simulink model "LHC_18kW_v8"  (R2015a)
settings: Solver=ode15s  StartTime=0.0  StopTime=1e4  RelTol=1e-3
libraries: simCryogenics_lib x152, nesl_utility x108, fl_lib x15
(part 1 of 2)
settings Model: Creator=SK248285  LastModifiedBy=FB229602
settings SimscapeCC: SimscapeLogType=all  SimscapeLogLimitData=off

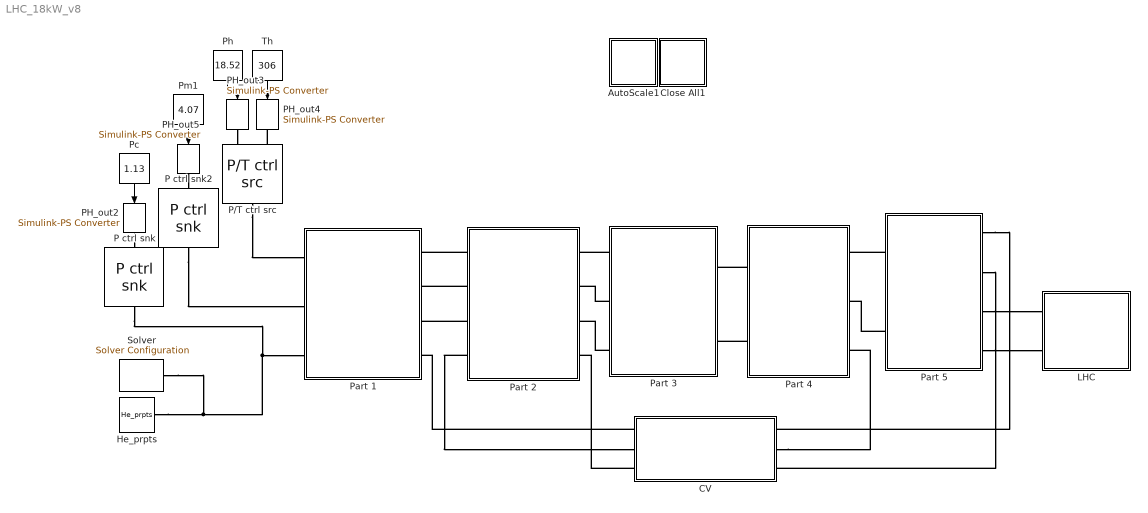
== system LHC_18kW_v8 ==
  AutoScale1 : Subsystem
      settings: OpenFcn=|
      | set(0, 'showhiddenhandles', 'on')
      | 
      | scope = findobj(0, 'Tag', 'SIMULINK_SIMSCOPE_FIGURE');
      | 
      | for i=1:length(scope)
      |   simscope('ScopeBar', 'ActionIcon', 'Find',     scope(i))
      | end
      | 
      | set(0, 'showhiddenhandles', 'off')
      mask Display: disp('Auto\nScale\nScope')
  CV : Subsystem
  Close All1 : Subsystem
      settings: OpenFcn=|
      | set(0, 'showhiddenhandles', 'on')
      | scope = findobj(0, 'Tag','SIMULINK_SIMSCOPE_FIGURE');
      | close(scope)
      | set(0, 'showhiddenhandles', 'off')
      mask Display: disp('Close\nAll\nScope')
  He_prpts : simCryogenics_lib/Utilities/He_prpts  P_min=0.01 bar  T_min=1.8 K  T_max=320 K  P_max=20 bar  Mol=4.0026 * 10 ^ (- 3) kg/mol
  LHC : Subsystem
  P ctrl snk : simCryogenics_lib/Sources_Sinks/P ctrl snk
  P ctrl snk2 : simCryogenics_lib/Sources_Sinks/P ctrl snk
  P/T ctrl src : simCryogenics_lib/Sources_Sinks/P//T ctrl src
  PH_out2 : nesl_utility/Simulink-PS Converter  PhysicalDomain=network_engine_domain  SubClassName=ps_input  LeftPortType=input  RightPortType=output  PseudoPeriodic=off  Frequencies=[]  NoiseDistribution=none  NoiseParameters=[]  Unit=bar  AffineConversion=off  InputFiltering=off  SimscapeFilterOrder=1  InputFilterTimeConstant=0.001  UdotUserProvided=1
  PH_out3 : nesl_utility/Simulink-PS Converter  PhysicalDomain=network_engine_domain  SubClassName=ps_input  LeftPortType=input  RightPortType=output  PseudoPeriodic=off  Frequencies=[]  NoiseDistribution=none  NoiseParameters=[]  Unit=bar  AffineConversion=off  InputFiltering=off  SimscapeFilterOrder=1  InputFilterTimeConstant=0.001  UdotUserProvided=1
  PH_out4 : nesl_utility/Simulink-PS Converter  PhysicalDomain=network_engine_domain  SubClassName=ps_input  LeftPortType=input  RightPortType=output  PseudoPeriodic=off  Frequencies=[]  NoiseDistribution=none  NoiseParameters=[]  Unit=K  AffineConversion=off  InputFiltering=off  SimscapeFilterOrder=1  InputFilterTimeConstant=0.001  UdotUserProvided=1
  PH_out5 : nesl_utility/Simulink-PS Converter  PhysicalDomain=network_engine_domain  SubClassName=ps_input  LeftPortType=input  RightPortType=output  PseudoPeriodic=off  Frequencies=[]  NoiseDistribution=none  NoiseParameters=[]  Unit=bar  AffineConversion=off  InputFiltering=off  SimscapeFilterOrder=1  InputFilterTimeConstant=0.001  UdotUserProvided=1
  Part 1 : Subsystem
  Part 2 : Subsystem
  Part 3 : Subsystem
  Part 4 : Subsystem
  Part 5 : Subsystem
  Pc : Constant  Value=1.13
  Ph : Constant  Value=18.52
  Pm1 : Constant  Value=4.07
  Solver : nesl_utility/Solver Configuration  PhysicalDomain=network_engine_domain  SubClassName=solver  LeftPortType=input  RightPortType=generic  Accelerate=off  Tones=[]  Harmonics=[]  SimulateNoise=off  Profile=off  UseLocalSampling=off  EnableSwitchedLinearOptims=on  FrequencyDomain=off  UseCCode=off  RelTol=0.001  AbsTol=1e-06  MinStep=1e-09  ToWorkspace=off  RevertToSquareIcSolve=off  NumHomotopyIterations=100  DoDC=off  ResidualTolerance=1e-09  UseLocalSolver=off  LocalSolverChoice=NE_BACKWARD_EULER_ADVANCER  LocalSolverSampleTime=0.001  DoFixedCost=off  MaxNonlinIter=3  MaxModeIter=2  LinearAlgebra=Sparse  DelaysMemoryBudget=1024  AutomaticFiltering=on  FilteringTimeConstant=0.001
  Th : Constant  Value=306
  wires:
  Th/1 -> PH_out4/1
  Ph/1 -> PH_out3/1
  Pc/1 -> PH_out2/1
  Pm1/1 -> PH_out5/1
  connections:
  PH_out3/RConn1 -- P/T ctrl src/LConn1
  P/T ctrl src/LConn2 -- PH_out4/RConn1
  PH_out2/RConn1 -- P ctrl snk/LConn1
  P/T ctrl src/RConn1 -- Part 1/LConn1
  PH_out5/RConn1 -- P ctrl snk2/LConn1
  P ctrl snk2/RConn1 -- Part 1/LConn2
  Solver/RConn1 -- He_prpts/RConn1 -- P ctrl snk/RConn1 -- Part 1/LConn3
  Part 2/LConn1 -- Part 1/RConn1
  Part 2/LConn2 -- Part 1/RConn2
  Part 2/LConn3 -- Part 1/RConn3
  Part 4/LConn1 -- Part 3/RConn1
  Part 4/LConn2 -- Part 3/RConn2
  Part 3/LConn1 -- Part 2/RConn1
  Part 3/LConn3 -- Part 2/RConn3
  Part 3/LConn2 -- Part 2/RConn2
  Part 5/LConn1 -- Part 4/RConn1
  Part 5/LConn2 -- Part 4/RConn2
  CV/LConn1 -- Part 1/RConn4
  Part 2/LConn4 -- CV/LConn2
  CV/LConn3 -- Part 2/RConn4
  CV/RConn2 -- Part 4/RConn3
  Part 5/RConn3 -- LHC/LConn1
  Part 5/RConn4 -- LHC/LConn2
  Part 5/RConn2 -- CV/RConn3
  Part 5/RConn1 -- CV/RConn1

== system LHC_18kW_v8/AutoScale1 ==

== system LHC_18kW_v8/CV ==
  CV236 : simCryogenics_lib/Elements/Valve  CVmax=0.92  ControlInputMin=0  ControlInputMax=100  Xt=0.65  Rv=50  lin_v=0  lim_v=0  K=2.4e-5 m^1.50000*kg^0.50000/s/bar^0.50000  Cmd_specify=off  Cmd_priority=High  Cmd=0  gamma_specify=off  gamma_priority=High  gamma=0  rho_specify=off  rho_priority=High  rho=0 kg/m^3  Xc_specify=off  Xc_priority=High  Xc=0  X_specify=off  X_priority=High  X=0  Y_specify=off  Y_priority=High  Y=0  CV_specify=off  CV_priority=High  CV=0
  CV293 : simCryogenics_lib/Elements/Valve  CVmax=289  ControlInputMin=0  ControlInputMax=100  Xt=0.65  Rv=50  lin_v=0  lim_v=0  K=2.4e-5 m^1.50000*kg^0.50000/s/bar^0.50000  Cmd_specify=off  Cmd_priority=High  Cmd=0  gamma_specify=off  gamma_priority=High  gamma=0  rho_specify=off  rho_priority=High  rho=0 kg/m^3  Xc_specify=off  Xc_priority=High  Xc=0  X_specify=off  X_priority=High  X=0  Y_specify=off  Y_priority=High  Y=0  CV_specify=off  CV_priority=High  CV=0
  CV294 : simCryogenics_lib/Elements/Valve  CVmax=450  ControlInputMin=0  ControlInputMax=100  Xt=0.65  Rv=50  lin_v=0  lim_v=0  K=2.4e-5 m^1.50000*kg^0.50000/s/bar^0.50000  Cmd_specify=off  Cmd_priority=High  Cmd=0  gamma_specify=off  gamma_priority=High  gamma=0  rho_specify=off  rho_priority=High  rho=0 kg/m^3  Xc_specify=off  Xc_priority=High  Xc=0  X_specify=off  X_priority=High  X=0  Y_specify=off  Y_priority=High  Y=0  CV_specify=off  CV_priority=High  CV=0
  CV299 : simCryogenics_lib/Elements/Valve  CVmax=185  ControlInputMin=0  ControlInputMax=100  Xt=0.65  Rv=50  lin_v=0  lim_v=0  K=2.4e-5 m^1.50000*kg^0.50000/s/bar^0.50000  Cmd_specify=off  Cmd_priority=High  Cmd=0  gamma_specify=off  gamma_priority=High  gamma=0  rho_specify=off  rho_priority=High  rho=0 kg/m^3  Xc_specify=off  Xc_priority=High  Xc=0  X_specify=off  X_priority=High  X=0  Y_specify=off  Y_priority=High  Y=0  CV_specify=off  CV_priority=High  CV=0
  Constant{2..5} (4 alike) : Constant  Value=0
  Distributor1 : simCryogenics_lib/Elements/Distributor2
  Distributor3 : simCryogenics_lib/Elements/Distributor2
  PH_out{1,6..8} (4 alike) : nesl_utility/Simulink-PS Converter  PhysicalDomain=network_engine_domain  SubClassName=ps_input  LeftPortType=input  RightPortType=output  PseudoPeriodic=off  Frequencies=[]  NoiseDistribution=none  NoiseParameters=[]  Unit=bar  AffineConversion=off  InputFiltering=off  SimscapeFilterOrder=1  InputFilterTimeConstant=0.001  UdotUserProvided=1
  V_in1 : PMIOPort  Port=1  Side=Right
  V_out4 : PMIOPort  Port=2  Side=Left
  V_out3 : PMIOPort  Port=3  Side=Left
  V_out2 : PMIOPort  Port=4  Side=Left
  V_out1 : PMIOPort  Port=5  Side=Right
  V_in2 : PMIOPort  Port=6  Side=Right
  wires:
  Constant2/1 -> PH_out1/1
  Constant5/1 -> PH_out8/1
  Constant3/1 -> PH_out6/1
  Constant4/1 -> PH_out7/1
  connections:
  V_out3/RConn1 -- CV236/RConn1
  PH_out1/RConn1 -- CV236/LConn1
  V_in1/RConn1 -- CV236/LConn2
  CV294/LConn2 -- Distributor3/RConn1
  CV299/RConn1 -- V_out4/RConn1
  CV299/LConn2 -- Distributor3/RConn2
  CV294/RConn1 -- V_out2/RConn1
  CV293/RConn1 -- V_out1/RConn1
  Distributor3/LConn1 -- Distributor1/RConn2
  PH_out8/RConn1 -- CV299/LConn1
  CV293/LConn2 -- Distributor1/RConn1
  Distributor1/LConn1 -- V_in2/RConn1
  PH_out6/RConn1 -- CV293/LConn1
  PH_out7/RConn1 -- CV294/LConn1

== system LHC_18kW_v8/Close All1 ==

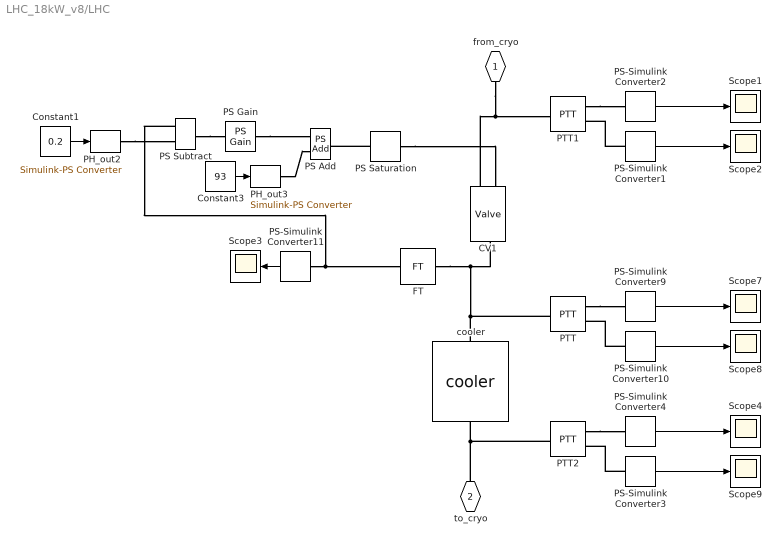
== system LHC_18kW_v8/LHC ==
  CV1 : simCryogenics_lib/Elements/Valve  CVmax=7  ControlInputMin=0  ControlInputMax=100  Xt=0.65  Rv=50  lin_v=0  lim_v=0  K=2.4e-5 m^1.50000*kg^0.50000/s/bar^0.50000  Cmd_specify=off  Cmd_priority=High  Cmd=0  gamma_specify=off  gamma_priority=High  gamma=0  rho_specify=off  rho_priority=High  rho=0 kg/m^3  Xc_specify=off  Xc_priority=High  Xc=0  X_specify=off  X_priority=High  X=0  Y_specify=off  Y_priority=High  Y=0  CV_specify=off  CV_priority=High  CV=0
  Constant1 : Constant  Value=0.2
  Constant3 : Constant  Value=93
  FT : simCryogenics_lib/Sensors/FT
  PH_out2 : nesl_utility/Simulink-PS Converter  PhysicalDomain=network_engine_domain  SubClassName=ps_input  LeftPortType=input  RightPortType=output  PseudoPeriodic=off  Frequencies=[]  NoiseDistribution=none  NoiseParameters=[]  Unit=bar  AffineConversion=off  InputFiltering=on  SimscapeFilterOrder=1  InputFilterTimeConstant=0.001  UdotUserProvided=1
  PH_out3 : nesl_utility/Simulink-PS Converter  PhysicalDomain=network_engine_domain  SubClassName=ps_input  LeftPortType=input  RightPortType=output  PseudoPeriodic=off  Frequencies=[]  NoiseDistribution=none  NoiseParameters=[]  Unit=bar  AffineConversion=off  InputFiltering=on  SimscapeFilterOrder=1  InputFilterTimeConstant=0.001  UdotUserProvided=1
  PS Add : fl_lib/Physical Signals/Functions/PS Add
  PS Gain : fl_lib/Physical Signals/Functions/PS Gain  gain=-200
  PS Saturation : fl_lib/Physical Signals/Nonlinear Operators/PS Saturation  upper_limit=100  lower_limit=0
  PS Subtract : fl_lib/Physical Signals/Functions/PS Subtract
  PS-Simulink Converter{1..4,9..11} (7 alike) : nesl_utility/PS-Simulink Converter  PhysicalDomain=network_engine_domain  SubClassName=ps_output  LeftPortType=input  RightPortType=output  PseudoPeriodic=off  Frequencies=[]  Unit=1  AffineConversion=off
  PTT : simCryogenics_lib/Sensors/PTT
  PTT1 : simCryogenics_lib/Sensors/PTT
  PTT2 : simCryogenics_lib/Sensors/PTT
  Scope{1..4,7..9} (7 alike) : Scope
      Scope1 settings: TimeRange=10000  SaveName=ScopeData9
      Scope2 settings: TimeRange=10000  SaveName=ScopeData4
      Scope3 settings: TimeRange=10000  YMin=0.672996  YMax=0.743838  SaveName=ScopeData66
      Scope4 settings: TimeRange=10000  SaveName=ScopeData10
      Scope7 settings: TimeRange=10000  SaveName=ScopeData2
      Scope8 settings: TimeRange=10000  SaveName=ScopeData3
      Scope9 settings: TimeRange=10000  SaveName=ScopeData8
  cooler : simCryogenics_lib/Utilities/cooler  Tout=4.6 K
  from_cryo : PMIOPort  Port=1  Side=Left
  to_cryo : PMIOPort  Port=2  Side=Left
  wires:
  PS-Simulink Converter2/1 -> Scope1/1
  PS-Simulink Converter9/1 -> Scope7/1
  PS-Simulink Converter10/1 -> Scope8/1
  PS-Simulink Converter1/1 -> Scope2/1
  PS-Simulink Converter3/1 -> Scope9/1
  PS-Simulink Converter4/1 -> Scope4/1
  PS-Simulink Converter11/1 -> Scope3/1
  Constant1/1 -> PH_out2/1
  Constant3/1 -> PH_out3/1
  connections:
  cooler/LConn1 -- PTT/LConn1 -- CV1/RConn1 -- FT/LConn1
  CV1/LConn2 -- from_cryo/RConn1 -- PTT1/LConn1
  PS-Simulink Converter10/LConn1 -- PTT/RConn2
  PS Saturation/RConn1 -- CV1/LConn1
  PS-Simulink Converter3/LConn1 -- PTT2/RConn2
  PTT2/RConn1 -- PS-Simulink Converter4/LConn1
  cooler/RConn1 -- PTT2/LConn1 -- to_cryo/RConn1
  PS-Simulink Converter1/LConn1 -- PTT1/RConn2
  PTT1/RConn1 -- PS-Simulink Converter2/LConn1
  PTT/RConn1 -- PS-Simulink Converter9/LConn1
  PS Subtract/LConn1 -- PS-Simulink Converter11/LConn1 -- FT/RConn1
  PS Saturation/LConn1 -- PS Add/RConn1
  PH_out2/RConn1 -- PS Subtract/LConn2
  PS Subtract/RConn1 -- PS Gain/LConn1
  PH_out3/RConn1 -- PS Add/LConn2
  PS Gain/RConn1 -- PS Add/LConn1

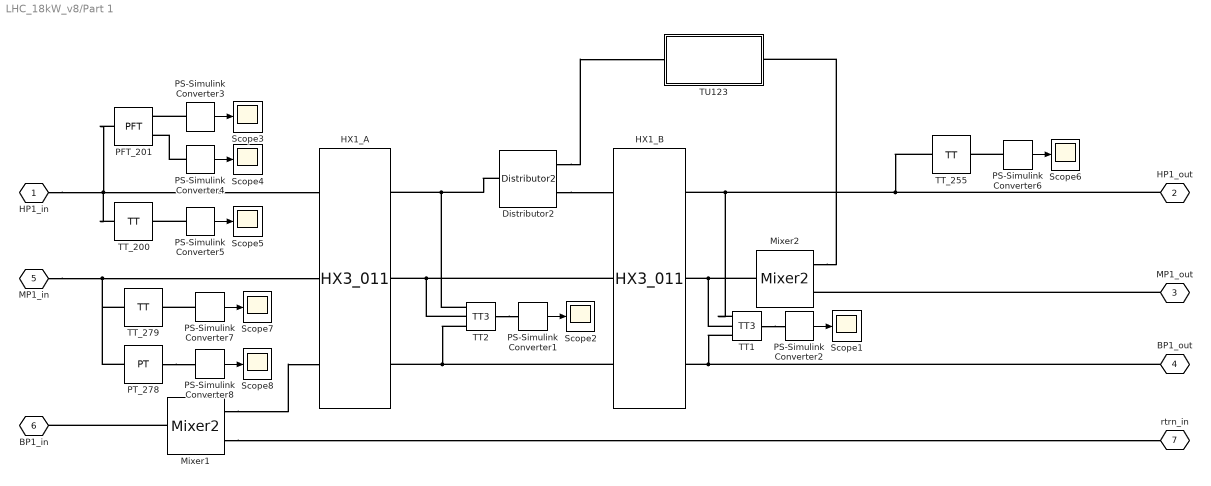
== system LHC_18kW_v8/Part 1 ==
  Distributor2 : simCryogenics_lib/Elements/Distributor2
  HX1_A : simCryogenics_lib/Elements/HX3_011  N=5  Vh=0.935 m^3  Vm=0.618 m^3  Vc=1.571 m^3  M=4593 kg  Kh=0.05 s*bar/kg  Km=0.025 s*bar/kg  Kc=0.0133 s*bar/kg  hh_m=316334 J/s/K  hh_c=316334 J/s/K  hm_c=1 J/s/K  Th0=306 K  Ph0=18.52 bar  Mh0=1.597 kg/s  Tm0=136 K  Pm0=4.07 bar  Mm0=0.8018 kg/s  Tc0=136 K  Pc0=1.05 bar  Mc0=0.7518 kg/s  sensh=0  sensm=1  sensc=1
  HX1_B : simCryogenics_lib/Elements/HX3_011  N=5  Vh=0.481 m^3  Vm=0.318 m^3  Vc=0.801 m^3  M=2366 kg  Kh=0.0586 s*bar/kg  Km=0.01247 s*bar/kg  Kc=0.0133 s*bar/kg  hh_m=119656 J/s/K  hh_c=112138 J/s/K  hm_c=1 J/s/K  Th0=143 K  Ph0=18.44 bar  Mh0=1.43 kg/s  Tm0=103 K  Pm0=4.09 bar  Mm0=0.8018 kg/s  Tc0=103 K  Pc0=1.135 bar  Mc0=0.7518 kg/s  sensh=0  sensm=1  sensc=1
  Mixer1 : simCryogenics_lib/Elements/Mixer2
  Mixer2 : simCryogenics_lib/Elements/Mixer2
  PFT_201 : simCryogenics_lib/Sensors/PFT
  PS-Simulink Converter{1..8} (8 alike) : nesl_utility/PS-Simulink Converter  PhysicalDomain=network_engine_domain  SubClassName=ps_output  LeftPortType=input  RightPortType=output  PseudoPeriodic=off  Frequencies=[]  Unit=1  AffineConversion=off
  PT_278 : simCryogenics_lib/Sensors/PT
  Scope{1..8} (8 alike) : Scope
      Scope1 settings: TimeRange=10000  SaveName=ScopeData3
      Scope2 settings: TimeRange=100000  YMin=100  YMax=400  SaveName=ScopeData11
      Scope3 settings: TimeRange=10000  SaveName=ScopeData23
      Scope4 settings: TimeRange=10000  YMin=1.85  YMax=1.8725  SaveName=ScopeData24
      Scope5 settings: TimeRange=10000  SaveName=ScopeData38
      Scope6 settings: TimeRange=10000  SaveName=ScopeData6
      Scope7 settings: TimeRange=10000  SaveName=ScopeData39
      Scope8 settings: TimeRange=10000  SaveName=ScopeData40
  TT1 : simCryogenics_lib/Sensors/TT3
  TT2 : simCryogenics_lib/Sensors/TT3
  TT_200 : simCryogenics_lib/Sensors/TT
  TT_255 : simCryogenics_lib/Sensors/TT
  TT_279 : simCryogenics_lib/Sensors/TT
  TU123 : Subsystem
  HP1_in : PMIOPort  Port=1  Side=Left
  HP1_out : PMIOPort  Port=2  Side=Right
  MP1_out : PMIOPort  Port=3  Side=Right
  BP1_out : PMIOPort  Port=4  Side=Right
  MP1_in : PMIOPort  Port=5  Side=Left
  BP1_in : PMIOPort  Port=6  Side=Left
  rtrn_in : PMIOPort  Port=7  Side=Right
  wires:
  PS-Simulink Converter1/1 -> Scope2/1
  PS-Simulink Converter2/1 -> Scope1/1
  PS-Simulink Converter3/1 -> Scope3/1
  PS-Simulink Converter4/1 -> Scope4/1
  PS-Simulink Converter5/1 -> Scope5/1
  PS-Simulink Converter7/1 -> Scope7/1
  PS-Simulink Converter8/1 -> Scope8/1
  PS-Simulink Converter6/1 -> Scope6/1
  connections:
  HX1_B/LConn1 -- TT2/LConn3 -- HX1_A/RConn1
  Distributor2/LConn1 -- TT2/LConn1 -- HX1_A/RConn3
  HX1_B/LConn2 -- TT2/LConn2 -- HX1_A/RConn2
  Distributor2/RConn2 -- HX1_B/LConn3
  BP1_out/RConn1 -- TT1/LConn3 -- HX1_B/RConn1
  MP1_out/RConn1 -- Mixer2/LConn1
  Mixer2/RConn1 -- TT1/LConn2 -- HX1_B/RConn2
  HP1_in/RConn1 -- HX1_A/LConn3 -- PFT_201/LConn1 -- TT_200/LConn1
  MP1_in/RConn1 -- PT_278/LConn1 -- TT_279/LConn1 -- HX1_A/LConn2
  Mixer1/LConn1 -- HX1_A/LConn1
  HP1_out/RConn1 -- TT_255/LConn1 -- TT1/LConn1 -- HX1_B/RConn3
  Distributor2/RConn1 -- TU123/LConn1
  Mixer2/LConn2 -- TU123/RConn1
  TT2/RConn1 -- PS-Simulink Converter1/LConn1
  TT1/RConn1 -- PS-Simulink Converter2/LConn1
  PS-Simulink Converter3/LConn1 -- PFT_201/RConn1
  PS-Simulink Converter4/LConn1 -- PFT_201/RConn2
  PS-Simulink Converter5/LConn1 -- TT_200/RConn1
  PS-Simulink Converter7/LConn1 -- TT_279/RConn1
  PT_278/RConn1 -- PS-Simulink Converter8/LConn1
  PS-Simulink Converter6/LConn1 -- TT_255/RConn1
  Mixer1/RConn1 -- BP1_in/RConn1
  Mixer1/LConn2 -- rtrn_in/RConn1

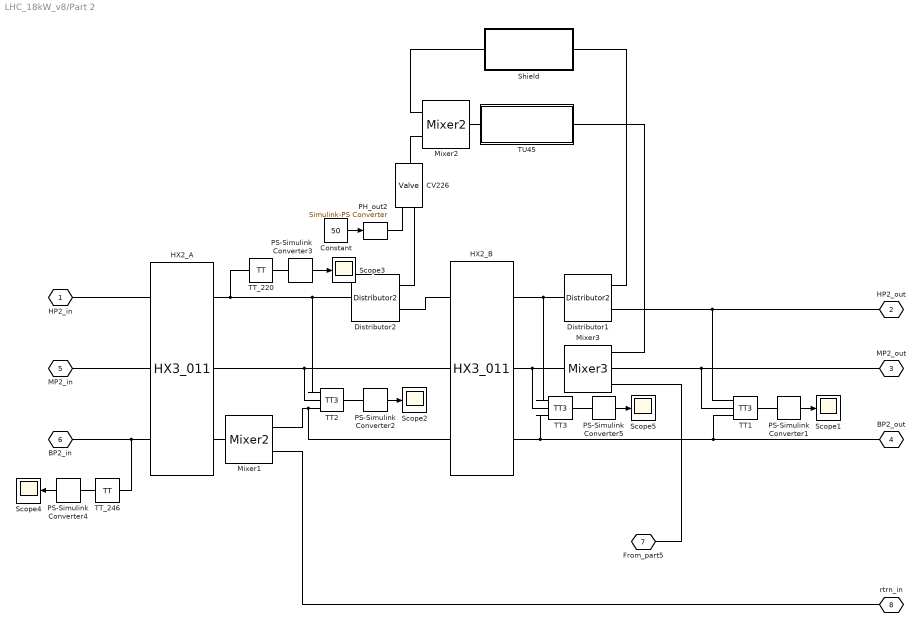
== system LHC_18kW_v8/Part 2 ==
  CV226 : simCryogenics_lib/Elements/Valve  CVmax=18.96  ControlInputMin=0  ControlInputMax=100  Xt=0.65  Rv=50  lin_v=0  lim_v=0  K=2.4e-5 m^1.50000*kg^0.50000/s/bar^0.50000  Cmd_specify=off  Cmd_priority=High  Cmd=0  gamma_specify=off  gamma_priority=High  gamma=0  rho_specify=off  rho_priority=High  rho=0 kg/m^3  Xc_specify=off  Xc_priority=High  Xc=0  X_specify=off  X_priority=High  X=0  Y_specify=off  Y_priority=High  Y=0  CV_specify=off  CV_priority=High  CV=0
  Constant : Constant  Value=50
  Distributor1 : simCryogenics_lib/Elements/Distributor2
  Distributor2 : simCryogenics_lib/Elements/Distributor2
  HX2_A : simCryogenics_lib/Elements/HX3_011  N=5  Vh=0.313 m^3  Vm=0.182 m^3  Vc=0.637 m^3  M=1697 kg  Kh=0.02198 s*bar/kg  Km=0.01754 s*bar/kg  Kc=0.01330 s*bar/kg  hh_m=111457 J/s/K  hh_c=146800 J/s/K  hm_c=1 J/s/K  Th0=94 K  Ph0=18.36 bar  Mh0=1.365 kg/s  Tm0=67 K  Pm0=4.1 bar  Mm0=0.57 kg/s  Tc0=67 K  Pc0=1.14 bar  Mc0=0.7518 kg/s  sensh=0  sensm=1  sensc=1
  HX2_B : simCryogenics_lib/Elements/HX3_011  N=5  Vh=0.344 m^3  Vm=0.182 m^3  Vc=0.637 m^3  M=1838 kg  Kh=0.02489 s*bar/kg  Km=0.01754 s*bar/kg  Kc=0.01330 s*bar/kg  hh_m=106764 J/s/K  hh_c=140360 J/s/K  hm_c=1 J/s/K  Th0=68.99 K  Ph0=18.33 bar  Mh0=1.205 kg/s  Tm0=49 K  Pm0=4.11 bar  Mm0=0.57 kg/s  Tc0=49 K  Pc0=1.15 bar  Mc0=0.7518 kg/s  sensh=0  sensm=1  sensc=1
  Mixer1 : simCryogenics_lib/Elements/Mixer2
  Mixer2 : simCryogenics_lib/Elements/Mixer2
  Mixer3 : simCryogenics_lib/Elements/Mixer3
  PH_out2 : nesl_utility/Simulink-PS Converter  PhysicalDomain=network_engine_domain  SubClassName=ps_input  LeftPortType=input  RightPortType=output  PseudoPeriodic=off  Frequencies=[]  NoiseDistribution=none  NoiseParameters=[]  Unit=bar  AffineConversion=off  InputFiltering=off  SimscapeFilterOrder=1  InputFilterTimeConstant=0.001  UdotUserProvided=1
  PS-Simulink Converter{1..5} (5 alike) : nesl_utility/PS-Simulink Converter  PhysicalDomain=network_engine_domain  SubClassName=ps_output  LeftPortType=input  RightPortType=output  PseudoPeriodic=off  Frequencies=[]  Unit=1  AffineConversion=off
  Scope{1..5} (5 alike) : Scope
      Scope1 settings: TimeRange=10000  SaveName=ScopeData17
      Scope2 settings: TimeRange=10000  SaveName=ScopeData12
      Scope3 settings: TimeRange=10000  SaveName=ScopeData10
      Scope4 settings: TimeRange=10000  SaveName=ScopeData42
      Scope5 settings: TimeRange=10000  SaveName=ScopeData65
  Shield : Subsystem
  TT1 : simCryogenics_lib/Sensors/TT3
  TT2 : simCryogenics_lib/Sensors/TT3
  TT3 : simCryogenics_lib/Sensors/TT3
  TT_220 : simCryogenics_lib/Sensors/TT
  TT_246 : simCryogenics_lib/Sensors/TT
  TU45 : Subsystem
  HP2_in : PMIOPort  Port=1  Side=Left
  HP2_out : PMIOPort  Port=2  Side=Right
  MP2_out : PMIOPort  Port=3  Side=Right
  BP2_out : PMIOPort  Port=4  Side=Right
  MP2_in : PMIOPort  Port=5  Side=Left
  BP2_in : PMIOPort  Port=6  Side=Left
  From_part5 : PMIOPort  Port=7  Side=Left
  rtrn_in : PMIOPort  Port=8  Side=Right
  wires:
  Constant/1 -> PH_out2/1
  PS-Simulink Converter1/1 -> Scope1/1
  PS-Simulink Converter2/1 -> Scope2/1
  PS-Simulink Converter4/1 -> Scope4/1
  PS-Simulink Converter3/1 -> Scope3/1
  PS-Simulink Converter5/1 -> Scope5/1
  connections:
  Distributor2/LConn1 -- TT2/LConn1 -- TT_220/LConn1 -- HX2_A/RConn3
  Distributor2/RConn1 -- CV226/LConn2
  CV226/LConn1 -- PH_out2/RConn1
  Distributor2/RConn2 -- HX2_B/LConn3
  HX2_B/LConn2 -- TT2/LConn2 -- HX2_A/RConn2
  TT2/LConn3 -- HX2_B/LConn1 -- Mixer1/LConn1
  Mixer2/LConn2 -- CV226/RConn1
  HX2_B/RConn3 -- TT3/LConn1 -- Distributor1/LConn1
  HP2_out/RConn1 -- Distributor1/RConn2 -- TT1/LConn1
  TT3/LConn2 -- Mixer3/RConn1 -- HX2_B/RConn2
  MP2_out/RConn1 -- TT1/LConn2 -- Mixer3/LConn2
  BP2_out/RConn1 -- TT3/LConn3 -- HX2_B/RConn1 -- TT1/LConn3
  HP2_in/RConn1 -- HX2_A/LConn3
  MP2_in/RConn1 -- HX2_A/LConn2
  BP2_in/RConn1 -- TT_246/LConn1 -- HX2_A/LConn1
  Shield/RConn1 -- Mixer2/LConn1
  Shield/LConn1 -- Distributor1/RConn1
  Mixer2/RConn1 -- TU45/LConn1
  TU45/RConn1 -- Mixer3/LConn1
  TT1/RConn1 -- PS-Simulink Converter1/LConn1
  TT2/RConn1 -- PS-Simulink Converter2/LConn1
  PS-Simulink Converter4/LConn1 -- TT_246/RConn1
  PS-Simulink Converter3/LConn1 -- TT_220/RConn1
  TT3/RConn1 -- PS-Simulink Converter5/LConn1
  Mixer3/LConn3 -- From_part5/RConn1
  Mixer1/RConn1 -- HX2_A/RConn1
  rtrn_in/RConn1 -- Mixer1/LConn2

== system LHC_18kW_v8/Part 3 ==
  Distributor2 : simCryogenics_lib/Elements/Distributor2
  HX3_A : simCryogenics_lib/Elements/HX3_011  N=5  Vh=0.113 m^3  Vm=0.054 m^3  Vc=0.463 m^3  M=995 kg  Kh=0.0520 s*bar/kg  Km=0.0607 s*bar/kg  Kc=0.0133 s*bar/kg  hh_m=23169 J/s/K  hh_c=105066 J/s/K  hm_c=1 J/s/K  Th0=48 K  Ph0=18.3 bar  Mh0=0.96 kg/s  Tm0=37 K  Pm0=4.12 bar  Mm0=0.1647 kg/s  Tc0=37 K  Pc0=1.153 bar  Mc0=0.7518 kg/s  sensh=0  sensm=1  sensc=1
  HX3_B : simCryogenics_lib/Elements/HX3_011  N=5  Vh=0.135 m^3  Vm=0.06 N*m/bar  Vc=0.553 m^3  M=1188 kg  Kh=0.03143 s*bar/kg  Km=0.12143 s*bar/kg  Kc=0.01330 s*bar/kg  hh_m=19406 J/s/K  hh_c=128682 J/s/K  hm_c=1 J/s/K  Th0=38 K  Ph0=18.25 bar  Mh0=0.7953 kg/s  Tm0=37 K  Pm0=4.13 bar  Mm0=0.1647 kg/s  Tc0=30 K  Pc0=1.158 bar  Mc0=0.7518 kg/s  sensh=0  sensm=1  sensc=1
  PS-Simulink Converter1 : nesl_utility/PS-Simulink Converter  PhysicalDomain=network_engine_domain  SubClassName=ps_output  LeftPortType=input  RightPortType=output  PseudoPeriodic=off  Frequencies=[]  Unit=1  AffineConversion=off
  PS-Simulink Converter6 : nesl_utility/PS-Simulink Converter  PhysicalDomain=network_engine_domain  SubClassName=ps_output  LeftPortType=input  RightPortType=output  PseudoPeriodic=off  Frequencies=[]  Unit=1  AffineConversion=off
  Scope1 : Scope
      settings: TimeRange=10000  SaveName=ScopeData21
  Scope6 : Scope
      settings: TimeRange=10000  SaveName=ScopeData25
  TT1 : simCryogenics_lib/Sensors/TT3
  TT7 : simCryogenics_lib/Sensors/TT3
  TU67 : Subsystem
  HP3_in : PMIOPort  Port=1  Side=Left
  HP3_out : PMIOPort  Port=2  Side=Right
  BP3_out : PMIOPort  Port=3  Side=Right
  MP3_in : PMIOPort  Port=4  Side=Left
  BP3_in : PMIOPort  Port=5  Side=Left
  wires:
  PS-Simulink Converter1/1 -> Scope1/1
  PS-Simulink Converter6/1 -> Scope6/1
  connections:
  BP3_in/RConn1 -- HX3_A/LConn1
  MP3_in/RConn1 -- HX3_A/LConn2
  HP3_in/RConn1 -- HX3_A/LConn3
  BP3_out/RConn1 -- TT1/LConn3 -- HX3_B/RConn1
  HP3_out/RConn1 -- TT1/LConn1 -- HX3_B/RConn3
  HX3_B/LConn1 -- TT7/LConn3 -- HX3_A/RConn1
  HX3_B/LConn2 -- TT7/LConn2 -- HX3_A/RConn2
  Distributor2/RConn2 -- HX3_B/LConn3
  Distributor2/LConn1 -- TT7/LConn1 -- HX3_A/RConn3
  TU67/RConn1 -- HX3_B/RConn2 -- TT1/LConn2
  Distributor2/RConn1 -- TU67/LConn1
  TT7/RConn1 -- PS-Simulink Converter1/LConn1
  TT1/RConn1 -- PS-Simulink Converter6/LConn1

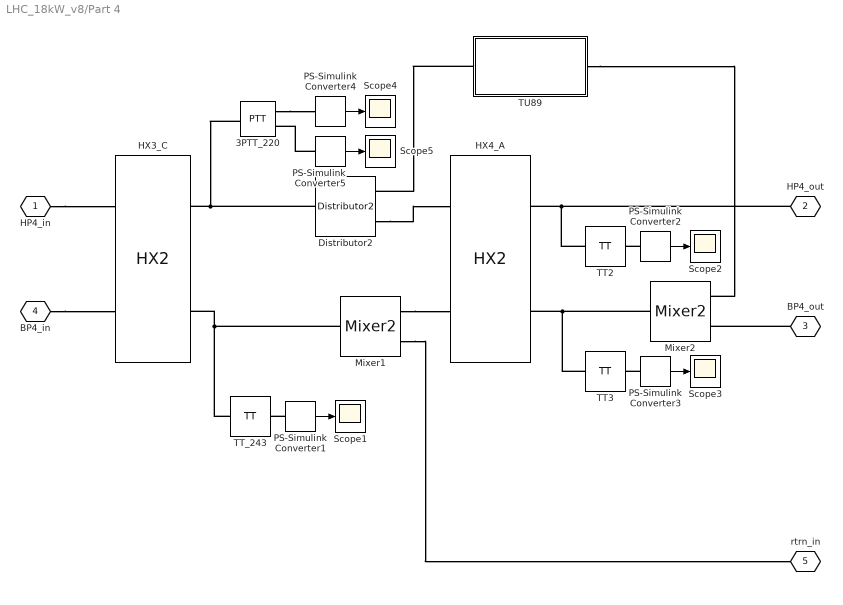
== system LHC_18kW_v8/Part 4 ==
  3PTT_220 : simCryogenics_lib/Sensors/PTT
  Distributor2 : simCryogenics_lib/Elements/Distributor2
  HX3_C : simCryogenics_lib/Elements/HX2  N=3  Vh=0.066 m^3  Vc=0.27 m^3  M=580 kg  Kh=0.0062869 s*bar/kg  Kc=0.0066507 s*bar/kg  h=66915 J/s/K  Th0=25 K  Ph0=18.225 bar  Mc0=0.7953 kg/s  Tc0=20 K  Pc0=1.16 bar  Mh0=0.7518 kg/s
  HX4_A : simCryogenics_lib/Elements/HX2  N=3  Vh=0.283 m^3  Vc=0.519 m^3  M=1821 kg  Kh=0.0121212 s*bar/kg  Kc=0.0073233 s*bar/kg  h=123127 J/s/K  Th0=21 K  Ph0=18.22 bar  Mc0=0.4125 kg/s  Tc0=9 K  Pc0=1.165 bar  Mh0=0.5462 kg/s
  Mixer1 : simCryogenics_lib/Elements/Mixer2
  Mixer2 : simCryogenics_lib/Elements/Mixer2
  PS-Simulink Converter{1..5} (5 alike) : nesl_utility/PS-Simulink Converter  PhysicalDomain=network_engine_domain  SubClassName=ps_output  LeftPortType=input  RightPortType=output  PseudoPeriodic=off  Frequencies=[]  Unit=1  AffineConversion=off
  Scope{1..5} (5 alike) : Scope
      Scope1 settings: TimeRange=10000  SaveName=ScopeData29
      Scope2 settings: TimeRange=10000  SaveName=ScopeData30
      Scope3 settings: TimeRange=10000  SaveName=ScopeData31
      Scope4 settings: TimeRange=10000  SaveName=ScopeData28
      Scope5 settings: TimeRange=10000  SaveName=ScopeData44
  TT2 : simCryogenics_lib/Sensors/TT
  TT3 : simCryogenics_lib/Sensors/TT
  TT_243 : simCryogenics_lib/Sensors/TT
  TU89 : Subsystem
  HP4_in : PMIOPort  Port=1  Side=Left
  HP4_out : PMIOPort  Port=2  Side=Right
  BP4_out : PMIOPort  Port=3  Side=Right
  BP4_in : PMIOPort  Port=4  Side=Left
  rtrn_in : PMIOPort  Port=5  Side=Right
  wires:
  PS-Simulink Converter1/1 -> Scope1/1
  PS-Simulink Converter2/1 -> Scope2/1
  PS-Simulink Converter3/1 -> Scope3/1
  PS-Simulink Converter4/1 -> Scope4/1
  PS-Simulink Converter5/1 -> Scope5/1
  connections:
  HP4_in/RConn1 -- HX3_C/LConn2
  BP4_in/RConn1 -- HX3_C/LConn1
  Distributor2/LConn1 -- 3PTT_220/LConn1 -- HX3_C/RConn2
  Distributor2/RConn2 -- HX4_A/LConn2
  TT_243/LConn1 -- HX3_C/RConn1 -- Mixer1/RConn1
  Mixer2/RConn1 -- TT3/LConn1 -- HX4_A/RConn1
  BP4_out/RConn1 -- Mixer2/LConn2
  HP4_out/RConn1 -- TT2/LConn1 -- HX4_A/RConn2
  PS-Simulink Converter1/LConn1 -- TT_243/RConn1
  PS-Simulink Converter2/LConn1 -- TT2/RConn1
  PS-Simulink Converter3/LConn1 -- TT3/RConn1
  TU89/LConn1 -- Distributor2/RConn1
  TU89/RConn1 -- Mixer2/LConn1
  3PTT_220/RConn1 -- PS-Simulink Converter4/LConn1
  PS-Simulink Converter5/LConn1 -- 3PTT_220/RConn2
  Mixer1/LConn1 -- HX4_A/LConn1
  Mixer1/LConn2 -- rtrn_in/RConn1

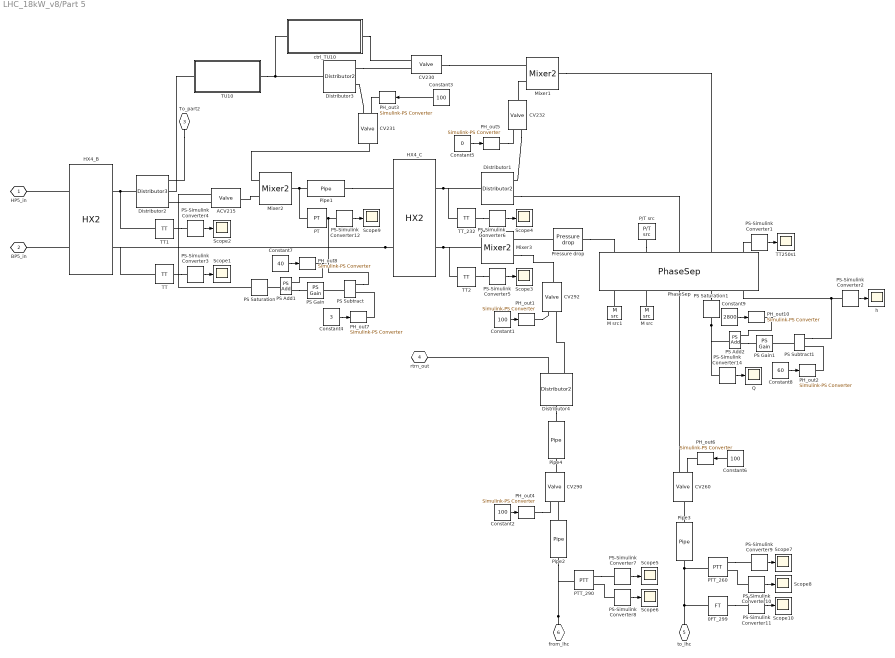
== system LHC_18kW_v8/Part 5 ==
  0FT_299 : simCryogenics_lib/Sensors/FT
  ACV215 : simCryogenics_lib/Elements/Valve  CVmax=8.1  ControlInputMin=0  ControlInputMax=100  Xt=0.65  Rv=50  lin_v=0  lim_v=0  K=2.4e-5 m^1.50000*kg^0.50000/s/bar^0.50000  Cmd_specify=off  Cmd_priority=High  Cmd=0  gamma_specify=off  gamma_priority=High  gamma=0  rho_specify=off  rho_priority=High  rho=0 kg/m^3  Xc_specify=off  Xc_priority=High  Xc=0  X_specify=off  X_priority=High  X=0  Y_specify=off  Y_priority=High  Y=0  CV_specify=off  CV_priority=High  CV=0
  CV230 : simCryogenics_lib/Elements/Valve  CVmax=8.1  ControlInputMin=0  ControlInputMax=100  Xt=0.65  Rv=50  lin_v=0  lim_v=0  K=2.4e-5 m^1.50000*kg^0.50000/s/bar^0.50000  Cmd_specify=off  Cmd_priority=High  Cmd=0  gamma_specify=off  gamma_priority=High  gamma=0  rho_specify=off  rho_priority=High  rho=0 kg/m^3  Xc_specify=off  Xc_priority=High  Xc=0  X_specify=off  X_priority=High  X=0  Y_specify=off  Y_priority=High  Y=0  CV_specify=off  CV_priority=High  CV=0
  CV231 : simCryogenics_lib/Elements/Valve  CVmax=52  ControlInputMin=0  ControlInputMax=100  Xt=0.65  Rv=50  lin_v=0  lim_v=0  K=2.4e-5 m^1.50000*kg^0.50000/s/bar^0.50000  Cmd_specify=off  Cmd_priority=High  Cmd=0  gamma_specify=off  gamma_priority=High  gamma=0  rho_specify=off  rho_priority=High  rho=0 kg/m^3  Xc_specify=off  Xc_priority=High  Xc=0  X_specify=off  X_priority=High  X=0  Y_specify=off  Y_priority=High  Y=0  CV_specify=off  CV_priority=High  CV=0
  CV232 : simCryogenics_lib/Elements/Valve  CVmax=8.1  ControlInputMin=0  ControlInputMax=100  Xt=0.65  Rv=50  lin_v=0  lim_v=0  K=2.4e-5 m^1.50000*kg^0.50000/s/bar^0.50000  Cmd_specify=off  Cmd_priority=High  Cmd=0  gamma_specify=off  gamma_priority=High  gamma=0  rho_specify=off  rho_priority=High  rho=0 kg/m^3  Xc_specify=off  Xc_priority=High  Xc=0  X_specify=off  X_priority=High  X=0  Y_specify=off  Y_priority=High  Y=0  CV_specify=off  CV_priority=High  CV=0
  CV260 : simCryogenics_lib/Elements/Valve  CVmax=96  ControlInputMin=0  ControlInputMax=100  Xt=0.65  Rv=50  lin_v=0  lim_v=0  K=2.4e-5 m^1.50000*kg^0.50000/s/bar^0.50000  Cmd_specify=off  Cmd_priority=High  Cmd=0  gamma_specify=off  gamma_priority=High  gamma=0  rho_specify=off  rho_priority=High  rho=0 kg/m^3  Xc_specify=off  Xc_priority=High  Xc=0  X_specify=off  X_priority=High  X=0  Y_specify=off  Y_priority=High  Y=0  CV_specify=off  CV_priority=High  CV=0
  CV290 : simCryogenics_lib/Elements/Valve  CVmax=428  ControlInputMin=0  ControlInputMax=100  Xt=0.65  Rv=50  lin_v=0  lim_v=0  K=2.4e-5 m^1.50000*kg^0.50000/s/bar^0.50000  Cmd_specify=off  Cmd_priority=High  Cmd=0  gamma_specify=off  gamma_priority=High  gamma=0  rho_specify=off  rho_priority=High  rho=0 kg/m^3  Xc_specify=off  Xc_priority=High  Xc=0  X_specify=off  X_priority=High  X=0  Y_specify=off  Y_priority=High  Y=0  CV_specify=off  CV_priority=High  CV=0
  CV292 : simCryogenics_lib/Elements/Valve  CVmax=113  ControlInputMin=0  ControlInputMax=100  Xt=0.65  Rv=50  lin_v=0  lim_v=0  K=2.4e-5 m^1.50000*kg^0.50000/s/bar^0.50000  Cmd_specify=off  Cmd_priority=High  Cmd=0  gamma_specify=off  gamma_priority=High  gamma=0  rho_specify=off  rho_priority=High  rho=0 kg/m^3  Xc_specify=off  Xc_priority=High  Xc=0  X_specify=off  X_priority=High  X=0  Y_specify=off  Y_priority=High  Y=0  CV_specify=off  CV_priority=High  CV=0
  Constant{1..3,6} (4 alike) : Constant  Value=100
  Constant4 : Constant  Value=3
  Constant5 : Constant  Value=0
  Constant7 : Constant  Value=40
  Constant8 : Constant  Value=60
  Constant9 : Constant  Value=2800
  Distributor1 : simCryogenics_lib/Elements/Distributor2
  Distributor2 : simCryogenics_lib/Elements/Distributor3
  Distributor3 : simCryogenics_lib/Elements/Distributor2
  Distributor4 : simCryogenics_lib/Elements/Distributor2
  HX4_B : simCryogenics_lib/Elements/HX2  N=3  Vh=0.057 m^3  Vc=0.094 m^3  M=398 kg  Kh=0.03636 s*bar/kg  Kc=0.00306 s*bar/kg  h=10308 J/s/K  Th0=9 K  Ph0=18.215 bar  Mc0=0.4125 kg/s  Tc0=6 K  Pc0=1.18 bar  Mh0=0.1634 kg/s
  HX4_C : simCryogenics_lib/Elements/HX2  N=3  Vh=0.043 m^3  Vc=0.094 m^3  M=274 kg  Kh=0.04014 s*bar/kg  Kc=0.00306 s*bar/kg  h=7776 J/s/K  Th0=7 K  Ph0=3.03 bar  Mc0=0.2491 kg/s  Tc0=5.5 K  Pc0=1.19 bar  Mh0=0.1634 kg/s
  M src : simCryogenics_lib/Sources_Sinks/M src  M=0 kg/s
  M src1 : simCryogenics_lib/Sources_Sinks/M src  M=0 kg/s
  Mixer1 : simCryogenics_lib/Elements/Mixer2
  Mixer2 : simCryogenics_lib/Elements/Mixer2
  Mixer3 : simCryogenics_lib/Elements/Mixer2
  P/T src : simCryogenics_lib/Sources_Sinks/P//T src  P=1 bar  T=300 K
  PH_out{1,3..6} (5 alike) : nesl_utility/Simulink-PS Converter  PhysicalDomain=network_engine_domain  SubClassName=ps_input  LeftPortType=input  RightPortType=output  PseudoPeriodic=off  Frequencies=[]  NoiseDistribution=none  NoiseParameters=[]  Unit=bar  AffineConversion=off  InputFiltering=off  SimscapeFilterOrder=1  InputFilterTimeConstant=0.001  UdotUserProvided=1
  PH_out{2,7..8,10} (4 alike) : nesl_utility/Simulink-PS Converter  PhysicalDomain=network_engine_domain  SubClassName=ps_input  LeftPortType=input  RightPortType=output  PseudoPeriodic=off  Frequencies=[]  NoiseDistribution=none  NoiseParameters=[]  Unit=bar  AffineConversion=off  InputFiltering=on  SimscapeFilterOrder=1  InputFilterTimeConstant=0.001  UdotUserProvided=1
  PS Add1 : fl_lib/Physical Signals/Functions/PS Add
  PS Add2 : fl_lib/Physical Signals/Functions/PS Add
  PS Gain : fl_lib/Physical Signals/Functions/PS Gain  gain=-200
  PS Gain1 : fl_lib/Physical Signals/Functions/PS Gain  gain=200
  PS Saturation : fl_lib/Physical Signals/Nonlinear Operators/PS Saturation  upper_limit=100  lower_limit=0
  PS Saturation1 : fl_lib/Physical Signals/Nonlinear Operators/PS Saturation  upper_limit=inf  lower_limit=0
  PS Subtract : fl_lib/Physical Signals/Functions/PS Subtract
  PS Subtract1 : fl_lib/Physical Signals/Functions/PS Subtract
  PS-Simulink Converter{1..12,14} (13 alike) : nesl_utility/PS-Simulink Converter  PhysicalDomain=network_engine_domain  SubClassName=ps_output  LeftPortType=input  RightPortType=output  PseudoPeriodic=off  Frequencies=[]  Unit=1  AffineConversion=off
  PT : simCryogenics_lib/Sensors/PT
  PTT_260 : simCryogenics_lib/Sensors/PTT
  PTT_290 : simCryogenics_lib/Sensors/PTT
  PhaseSep : simCryogenics_lib/Elements/PhaseSep  Ideal1=1  DeltaT1=0.05 K  N1=10  h1=950.3318 W/K  Ideal2=1  DeltaT2=0.05 K  N2=10  h2=950.3318 W/K  hmax=2.1 m  S=0.9503 m^2  P0=1.25 bar  h0=50
  Pipe1 : simCryogenics_lib/Elements/Pipe  Vol=0.01 m^3  Ideal=0  P0=3.5 bar  T0=5.555 K
  Pipe2 : simCryogenics_lib/Elements/Pipe  Vol=0.01 m^3  Ideal=0  P0=1.3 bar  T0=20 K
  Pipe3 : simCryogenics_lib/Elements/Pipe  Vol=0.01 m^3  Ideal=0  P0=5 bar  T0=4.6 K
  Pipe4 : simCryogenics_lib/Elements/Pipe  Vol=0.01 m^3  Ideal=0  P0=1.25 bar  T0=20 K
  Pressure drop : simCryogenics_lib/Utilities/Pressure drop  K=0.01/0.2 s*bar/kg
  Q : Scope
      settings: TimeRange=10000  YMin=4929.77  YMax=5448.69  SaveName=TT3
  Scope{1..10} (10 alike) : Scope
      Scope1 settings: TimeRange=10000  SaveName=ScopeData18
      Scope10 settings: TimeRange=10000  SaveName=ScopeData51
      Scope2 settings: TimeRange=10000  SaveName=ScopeData19
      Scope3 settings: TimeRange=10000  SaveName=ScopeData20
      Scope4 settings: TimeRange=233  YMin=4.56167  YMax=4.56207  SaveName=ScopeData22
      Scope5 settings: TimeRange=10000  YMin=1.40029  YMax=1.40035  SaveName=ScopeData47
      Scope6 settings: TimeRange=2111.844735963061  YMin=4.58386  YMax=4.58391  SaveName=ScopeData48
      Scope7 settings: TimeRange=10000  SaveName=ScopeData49
      Scope8 settings: TimeRange=10000  SaveName=ScopeData50
      Scope9 settings: TimeRange=233  YMin=1.5  YMax=3.1
  TT : simCryogenics_lib/Sensors/TT
  TT1 : simCryogenics_lib/Sensors/TT
  TT2 : simCryogenics_lib/Sensors/TT
  TT250s1 : Scope
      settings: SaveName=TT1
  TT_232 : simCryogenics_lib/Sensors/TT
  TU10 : Subsystem
  ctrl_TU10 : Subsystem
  h : Scope
      settings: TimeRange=100000  YMin=67.1304  YMax=74.1968  SaveName=TT
  HP5_in : PMIOPort  Port=1  Side=Left
  BP5_in : PMIOPort  Port=2  Side=Left
  To_part2 : PMIOPort  Port=3  Side=Right
  rtrn_out : PMIOPort  Port=4  Side=Right
  to_lhc : PMIOPort  Port=5  Side=Right
  from_lhc : PMIOPort  Port=6  Side=Right
  wires:
  PS-Simulink Converter6/1 -> Scope4/1
  PS-Simulink Converter5/1 -> Scope3/1
  PS-Simulink Converter4/1 -> Scope2/1
  PS-Simulink Converter3/1 -> Scope1/1
  PS-Simulink Converter1/1 -> TT250s1/1
  Constant5/1 -> PH_out5/1
  Constant3/1 -> PH_out3/1
  Constant1/1 -> PH_out1/1
  PS-Simulink Converter12/1 -> Scope9/1
  Constant4/1 -> PH_out7/1
  Constant7/1 -> PH_out8/1
  PS-Simulink Converter11/1 -> Scope10/1
  PS-Simulink Converter10/1 -> Scope8/1
  PS-Simulink Converter9/1 -> Scope7/1
  PS-Simulink Converter8/1 -> Scope6/1
  PS-Simulink Converter7/1 -> Scope5/1
  Constant2/1 -> PH_out4/1
  Constant6/1 -> PH_out6/1
  PS-Simulink Converter2/1 -> h/1
  Constant8/1 -> PH_out2/1
  Constant9/1 -> PH_out10/1
  PS-Simulink Converter14/1 -> Q/1
  connections:
  TT_232/RConn1 -- PS-Simulink Converter6/LConn1
  TT2/RConn1 -- PS-Simulink Converter5/LConn1
  TT1/RConn1 -- PS-Simulink Converter4/LConn1
  TT/RConn1 -- PS-Simulink Converter3/LConn1
  TU10/LConn1 -- Distributor2/RConn2
  TU10/RConn1 -- ctrl_TU10/LConn1 -- Distributor3/LConn1
  Pressure drop/LConn1 -- PhaseSep/LConn1
  M src1/RConn1 -- PhaseSep/RConn1
  PS-Simulink Converter1/LConn1 -- PhaseSep/LConn5
  M src/RConn1 -- PhaseSep/RConn2
  P/T src/RConn1 -- PhaseSep/LConn2
  Distributor1/RConn2 -- PhaseSep/LConn3
  Pipe1/RConn1 -- HX4_C/LConn2
  Pipe1/LConn1 -- PT/LConn1 -- Mixer2/RConn1
  Pressure drop/RConn1 -- Mixer3/LConn1
  HX4_C/RConn1 -- TT2/LConn1 -- Mixer3/RConn1
  Mixer1/RConn1 -- PhaseSep/LConn4
  Mixer1/LConn2 -- CV232/RConn1
  CV232/LConn2 -- Distributor1/RConn1
  PH_out5/RConn1 -- CV232/LConn1
  HX4_C/RConn2 -- TT_232/LConn1 -- Distributor1/LConn1
  Mixer2/LConn1 -- CV231/RConn1
  Distributor3/RConn1 -- CV230/LConn2
  CV230/RConn1 -- Mixer1/LConn1
  PH_out3/RConn1 -- CV231/LConn1
  CV231/LConn2 -- Distributor3/RConn2
  Mixer2/LConn2 -- ACV215/RConn1
  PS Saturation/RConn1 -- ACV215/LConn1
  ACV215/LConn2 -- Distributor2/RConn3
  HX4_B/LConn2 -- HP5_in/RConn1
  HX4_B/LConn1 -- BP5_in/RConn1
  HX4_C/LConn1 -- TT/LConn1 -- HX4_B/RConn1
  TT1/LConn1 -- Distributor2/LConn1 -- HX4_B/RConn2
  ctrl_TU10/RConn1 -- CV230/LConn1
  PH_out1/RConn1 -- CV292/LConn1
  Mixer3/LConn2 -- CV292/RConn1
  PS-Simulink Converter12/LConn1 -- PS Subtract/LConn1 -- PT/RConn1
  Distributor4/RConn2 -- CV292/LConn2
  Distributor4/RConn1 -- rtrn_out/RConn1
  To_part2/RConn1 -- Distributor2/RConn1
  PS Subtract/RConn1 -- PS Gain/LConn1
  PH_out8/RConn1 -- PS Add1/LConn1
  PS Add1/RConn1 -- PS Saturation/LConn1
  PS Add1/LConn2 -- PS Gain/RConn1
  PH_out7/RConn1 -- PS Subtract/LConn2
  to_lhc/RConn1 -- 0FT_299/LConn1 -- Pipe3/RConn1 -- PTT_260/LConn1
  from_lhc/RConn1 -- PTT_290/LConn1 -- Pipe2/LConn1
  PTT_260/RConn1 -- PS-Simulink Converter9/LConn1
  CV260/LConn2 -- PhaseSep/RConn3
  CV290/RConn1 -- Pipe4/LConn1
  PS-Simulink Converter10/LConn1 -- PTT_260/RConn2
  0FT_299/RConn1 -- PS-Simulink Converter11/LConn1
  Pipe2/RConn1 -- CV290/LConn2
  PTT_290/RConn1 -- PS-Simulink Converter7/LConn1
  PS-Simulink Converter8/LConn1 -- PTT_290/RConn2
  Pipe3/LConn1 -- CV260/RConn1
  PH_out6/RConn1 -- CV260/LConn1
  PH_out4/RConn1 -- CV290/LConn1
  Distributor4/LConn1 -- Pipe4/RConn1
  PS Saturation1/LConn1 -- PS Add2/RConn1 -- PS-Simulink Converter14/LConn1
  PS Subtract1/LConn1 -- PhaseSep/RConn5 -- PS-Simulink Converter2/LConn1
  PS Subtract1/RConn1 -- PS Gain1/LConn1
  PH_out2/RConn1 -- PS Subtract1/LConn2
  PH_out10/RConn1 -- PS Add2/LConn1
  PhaseSep/RConn4 -- PS Saturation1/RConn1
  PS Add2/LConn2 -- PS Gain1/RConn1

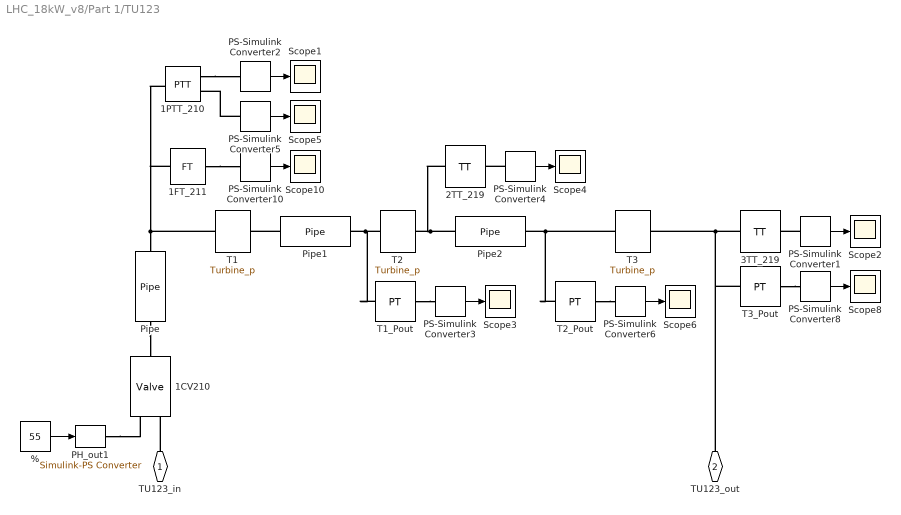
== system LHC_18kW_v8/Part 1/TU123 ==
  % : Constant  Value=55
  1CV210 : simCryogenics_lib/Elements/Valve  CVmax=26  ControlInputMin=0  ControlInputMax=100  Xt=0.65  Rv=50  lin_v=0  lim_v=0  K=2.4e-5 m^1.50000*kg^0.50000/s/bar^0.50000  Cmd_specify=off  Cmd_priority=High  Cmd=0  gamma_specify=off  gamma_priority=High  gamma=0  rho_specify=off  rho_priority=High  rho=0 kg/m^3  Xc_specify=off  Xc_priority=High  Xc=0  X_specify=off  X_priority=High  X=0  Y_specify=off  Y_priority=High  Y=0  CV_specify=off  CV_priority=High  CV=0
  1FT_211 : simCryogenics_lib/Sensors/FT
  1PTT_210 : simCryogenics_lib/Sensors/PTT
  2TT_219 : simCryogenics_lib/Sensors/TT
  3TT_219 : simCryogenics_lib/Sensors/TT
  PH_out1 : nesl_utility/Simulink-PS Converter  PhysicalDomain=network_engine_domain  SubClassName=ps_input  LeftPortType=input  RightPortType=output  PseudoPeriodic=off  Frequencies=[]  NoiseDistribution=none  NoiseParameters=[]  Unit=1  AffineConversion=off  InputFiltering=off  SimscapeFilterOrder=1  InputFilterTimeConstant=0.001  UdotUserProvided=1
  PS-Simulink Converter{1..6,8,10} (8 alike) : nesl_utility/PS-Simulink Converter  PhysicalDomain=network_engine_domain  SubClassName=ps_output  LeftPortType=input  RightPortType=output  PseudoPeriodic=off  Frequencies=[]  Unit=1  AffineConversion=off
  Pipe : simCryogenics_lib/Elements/Pipe  Vol=0.01 m^3  Ideal=0  P0=13.5 bar  T0=137 K
  Pipe1 : simCryogenics_lib/Elements/Pipe  Vol=0.01 m^3  Ideal=0  P0=9 bar  T0=132 K
  Pipe2 : simCryogenics_lib/Elements/Pipe  Vol=0.01 m^3  Ideal=0  P0=6 bar  T0=118 K
  Scope{1..6,8,10} (8 alike) : Scope
      Scope1 settings: TimeRange=10000  YMin=12.9332  YMax=12.9353  SaveName=ScopeData4
      Scope10 settings: TimeRange=10000
      Scope2 settings: TimeRange=10000  YMin=100  YMax=180  SaveName=ScopeData2
      Scope3 settings: TimeRange=10000  YMin=17  YMax=17.1  SaveName=ScopeData55
      Scope4 settings: TimeRange=10000  YMin=100  YMax=180  SaveName=ScopeData56
      Scope5 settings: TimeRange=10000  SaveName=ScopeData41
      Scope6 settings: TimeRange=10000  SaveName=ScopeData57
      Scope8 settings: TimeRange=10000
  T1 : simCryogenics_lib/Elements/Turbine_p  A=9.5063e-05 m^2  D=0.0296 m  Mass=1.8 kg  cst_eff=0  eta0=0.73  Tin0=137 K  Pin0=13 bar  Pout0=8.67 bar  N0=2500 1/s  Q0=0 W  v0=0  I=0 kg*m^2  gamma_specify=off  gamma_priority=High  gamma=0  C_specify=off  C_priority=High  C=0  Z_specify=off  Z_priority=High  Z=0  Cp_specify=off  Cp_priority=High  Cp=0 kJ/kg/K  Sin_specify=off  Sin_priority=High  Sin=0 kJ/kg  T_specify=off  T_priority=High  T=0 K  HoutIs_specify=off  HoutIs_priority=High  HoutIs=0 kJ/kg  u1_specify=off  u1_priority=High  u1=0 m/s  c1_specify=off  c1_priority=High  c1=0 m/s  v_specify=off  v_priority=High  v=0  eta_specify=off  eta_priority=High  eta=0  eta_var_specify=off  eta_var_priority=High  eta_var=0  N_specify=off  N_priority=High  N=0 rad/s  Q_specify=off  Q_priority=High  Q=0 W
  T1_Pout : simCryogenics_lib/Sensors/PT
  T2 : simCryogenics_lib/Elements/Turbine_p  A=1.3451e-04 m^2  D=0.0381 m  Mass=5.4 kg  cst_eff=0  eta0=0.75  Tin0=132 K  Pin0=9 bar  Pout0=6 bar  N0=1900 1/s  Q0=0 W  v0=0  I=0 kg*m^2  gamma_specify=off  gamma_priority=High  gamma=0  C_specify=off  C_priority=High  C=0  Z_specify=off  Z_priority=High  Z=0  Cp_specify=off  Cp_priority=High  Cp=0 kJ/kg/K  Sin_specify=off  Sin_priority=High  Sin=0 kJ/kg  T_specify=off  T_priority=High  T=0 K  HoutIs_specify=off  HoutIs_priority=High  HoutIs=0 kJ/kg  u1_specify=off  u1_priority=High  u1=0 m/s  c1_specify=off  c1_priority=High  c1=0 m/s  v_specify=off  v_priority=High  v=0  eta_specify=off  eta_priority=High  eta=0  eta_var_specify=off  eta_var_priority=High  eta_var=0  N_specify=off  N_priority=High  N=0 rad/s  Q_specify=off  Q_priority=High  Q=0 W
  T2_Pout : simCryogenics_lib/Sensors/PT
  T3 : simCryogenics_lib/Elements/Turbine_p  A=1.9050e-04 m^2  D=0.0471 m  Mass=5.4 kg  cst_eff=0  eta0=0.71  Tin0=118 K  Pin0=6 bar  Pout0=2.86 bar  N0=1900 1/s  Q0=0 W  v0=0  I=0 kg*m^2  gamma_specify=off  gamma_priority=High  gamma=0  C_specify=off  C_priority=High  C=0  Z_specify=off  Z_priority=High  Z=0  Cp_specify=off  Cp_priority=High  Cp=0 kJ/kg/K  Sin_specify=off  Sin_priority=High  Sin=0 kJ/kg  T_specify=off  T_priority=High  T=0 K  HoutIs_specify=off  HoutIs_priority=High  HoutIs=0 kJ/kg  u1_specify=off  u1_priority=High  u1=0 m/s  c1_specify=off  c1_priority=High  c1=0 m/s  v_specify=off  v_priority=High  v=0  eta_specify=off  eta_priority=High  eta=0  eta_var_specify=off  eta_var_priority=High  eta_var=0  N_specify=off  N_priority=High  N=0 rad/s  Q_specify=off  Q_priority=High  Q=0 W
  T3_Pout : simCryogenics_lib/Sensors/PT
  TU123_in : PMIOPort  Port=1  Side=Left
  TU123_out : PMIOPort  Port=2  Side=Right
  wires:
  %/1 -> PH_out1/1
  PS-Simulink Converter1/1 -> Scope2/1
  PS-Simulink Converter2/1 -> Scope1/1
  PS-Simulink Converter5/1 -> Scope5/1
  PS-Simulink Converter10/1 -> Scope10/1
  PS-Simulink Converter8/1 -> Scope8/1
  PS-Simulink Converter3/1 -> Scope3/1
  PS-Simulink Converter4/1 -> Scope4/1
  PS-Simulink Converter6/1 -> Scope6/1
  connections:
  TU123_in/RConn1 -- 1CV210/LConn2
  3TT_219/LConn1 -- T3_Pout/LConn1 -- TU123_out/RConn1 -- T3/RConn1
  T1/LConn1 -- 1PTT_210/LConn1 -- 1FT_211/LConn1 -- Pipe/RConn1
  Pipe/LConn1 -- 1CV210/RConn1
  PH_out1/RConn1 -- 1CV210/LConn1
  PS-Simulink Converter1/LConn1 -- 3TT_219/RConn1
  1PTT_210/RConn1 -- PS-Simulink Converter2/LConn1
  PS-Simulink Converter5/LConn1 -- 1PTT_210/RConn2
  1FT_211/RConn1 -- PS-Simulink Converter10/LConn1
  T3_Pout/RConn1 -- PS-Simulink Converter8/LConn1
  Pipe1/LConn1 -- T1/RConn1
  T2/LConn1 -- T1_Pout/LConn1 -- Pipe1/RConn1
  Pipe2/LConn1 -- 2TT_219/LConn1 -- T2/RConn1
  T3/LConn1 -- T2_Pout/LConn1 -- Pipe2/RConn1
  T1_Pout/RConn1 -- PS-Simulink Converter3/LConn1
  PS-Simulink Converter4/LConn1 -- 2TT_219/RConn1
  T2_Pout/RConn1 -- PS-Simulink Converter6/LConn1

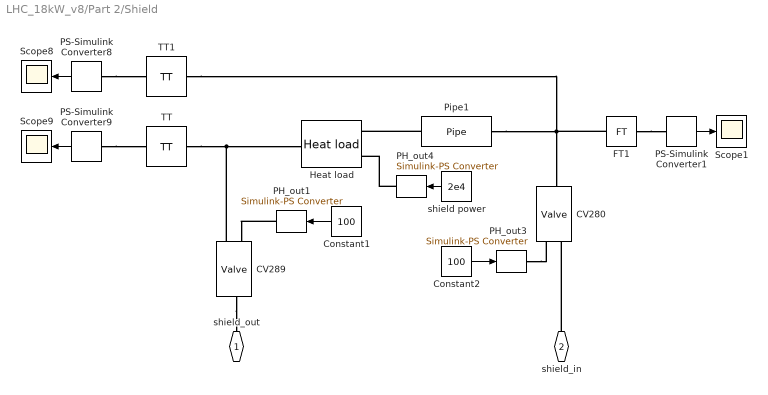
== system LHC_18kW_v8/Part 2/Shield ==
  CV280 : simCryogenics_lib/Elements/Valve  CVmax=63  ControlInputMin=0  ControlInputMax=100  Xt=0.65  Rv=50  lin_v=0  lim_v=0  K=2.4e-5 m^1.50000*kg^0.50000/s/bar^0.50000  Cmd_specify=off  Cmd_priority=High  Cmd=0  gamma_specify=off  gamma_priority=High  gamma=0  rho_specify=off  rho_priority=High  rho=0 kg/m^3  Xc_specify=off  Xc_priority=High  Xc=0  X_specify=off  X_priority=High  X=0  Y_specify=off  Y_priority=High  Y=0  CV_specify=off  CV_priority=High  CV=0
  CV289 : simCryogenics_lib/Elements/Valve  CVmax=113  ControlInputMin=0  ControlInputMax=100  Xt=0.65  Rv=50  lin_v=0  lim_v=0  K=2.4e-5 m^1.50000*kg^0.50000/s/bar^0.50000  Cmd_specify=off  Cmd_priority=High  Cmd=0  gamma_specify=off  gamma_priority=High  gamma=0  rho_specify=off  rho_priority=High  rho=0 kg/m^3  Xc_specify=off  Xc_priority=High  Xc=0  X_specify=off  X_priority=High  X=0  Y_specify=off  Y_priority=High  Y=0  CV_specify=off  CV_priority=High  CV=0
  Constant1 : Constant  Value=100
  Constant2 : Constant  Value=100
  FT1 : simCryogenics_lib/Sensors/FT
  Heat load : simCryogenics_lib/Utilities/Heat load
  PH_out1 : nesl_utility/Simulink-PS Converter  PhysicalDomain=network_engine_domain  SubClassName=ps_input  LeftPortType=input  RightPortType=output  PseudoPeriodic=off  Frequencies=[]  NoiseDistribution=none  NoiseParameters=[]  Unit=bar  AffineConversion=off  InputFiltering=off  SimscapeFilterOrder=1  InputFilterTimeConstant=0.001  UdotUserProvided=1
  PH_out3 : nesl_utility/Simulink-PS Converter  PhysicalDomain=network_engine_domain  SubClassName=ps_input  LeftPortType=input  RightPortType=output  PseudoPeriodic=off  Frequencies=[]  NoiseDistribution=none  NoiseParameters=[]  Unit=bar  AffineConversion=off  InputFiltering=off  SimscapeFilterOrder=1  InputFilterTimeConstant=0.001  UdotUserProvided=1
  PH_out4 : nesl_utility/Simulink-PS Converter  PhysicalDomain=network_engine_domain  SubClassName=ps_input  LeftPortType=input  RightPortType=output  PseudoPeriodic=off  Frequencies=[]  NoiseDistribution=none  NoiseParameters=[]  Unit=J/s  AffineConversion=off  InputFiltering=off  SimscapeFilterOrder=1  InputFilterTimeConstant=0.001  UdotUserProvided=1
  PS-Simulink Converter1 : nesl_utility/PS-Simulink Converter  PhysicalDomain=network_engine_domain  SubClassName=ps_output  LeftPortType=input  RightPortType=output  PseudoPeriodic=off  Frequencies=[]  Unit=1  AffineConversion=off
  PS-Simulink Converter8 : nesl_utility/PS-Simulink Converter  PhysicalDomain=network_engine_domain  SubClassName=ps_output  LeftPortType=input  RightPortType=output  PseudoPeriodic=off  Frequencies=[]  Unit=1  AffineConversion=off
  PS-Simulink Converter9 : nesl_utility/PS-Simulink Converter  PhysicalDomain=network_engine_domain  SubClassName=ps_output  LeftPortType=input  RightPortType=output  PseudoPeriodic=off  Frequencies=[]  Unit=1  AffineConversion=off
  Pipe1 : simCryogenics_lib/Elements/Pipe  Vol=1 m^3  Ideal=0  P0=17 bar  T0=90 K
  Scope1 : Scope
      settings: TimeRange=10000  SaveName=ScopeData8
  Scope8 : Scope
      settings: TimeRange=10000  SaveName=ScopeData14
  Scope9 : Scope
      settings: TimeRange=10000  SaveName=ScopeData15
  TT : simCryogenics_lib/Sensors/TT
  TT1 : simCryogenics_lib/Sensors/TT
  shield power : Constant  Value=2e4
  shield_out : PMIOPort  Port=1  Side=Right
  shield_in : PMIOPort  Port=2  Side=Left
  wires:
  Constant1/1 -> PH_out1/1
  Constant2/1 -> PH_out3/1
  shield power/1 -> PH_out4/1
  PS-Simulink Converter1/1 -> Scope1/1
  PS-Simulink Converter8/1 -> Scope8/1
  PS-Simulink Converter9/1 -> Scope9/1
  connections:
  CV289/RConn1 -- shield_out/RConn1
  PH_out1/RConn1 -- CV289/LConn1
  CV289/LConn2 -- TT/LConn1 -- Heat load/RConn1
  Pipe1/LConn1 -- FT1/LConn1 -- TT1/LConn1 -- CV280/RConn1
  PH_out3/RConn1 -- CV280/LConn1
  shield_in/RConn1 -- CV280/LConn2
  PH_out4/RConn1 -- Heat load/LConn2
  Pipe1/RConn1 -- Heat load/LConn1
  FT1/RConn1 -- PS-Simulink Converter1/LConn1
  PS-Simulink Converter8/LConn1 -- TT1/RConn1
  PS-Simulink Converter9/LConn1 -- TT/RConn1
